simulink model "mcs_sim"  (R2014a)
settings: Solver=ode45  StartTime=0.0  StopTime=0.1  RelTol=1e-3
values from neighbouring files (symbols this model uses):
  mcs_sys = sys_class    [create_all_sys.m]
  sysr = ss(A_r,B_r,C_r,0)    [model_reduction.m]
undefined symbols (not defined in the file or in its folder): sysb, sysb_x0, sysr_x0
settings Model: Creator=UX31  LastModifiedBy=UX31

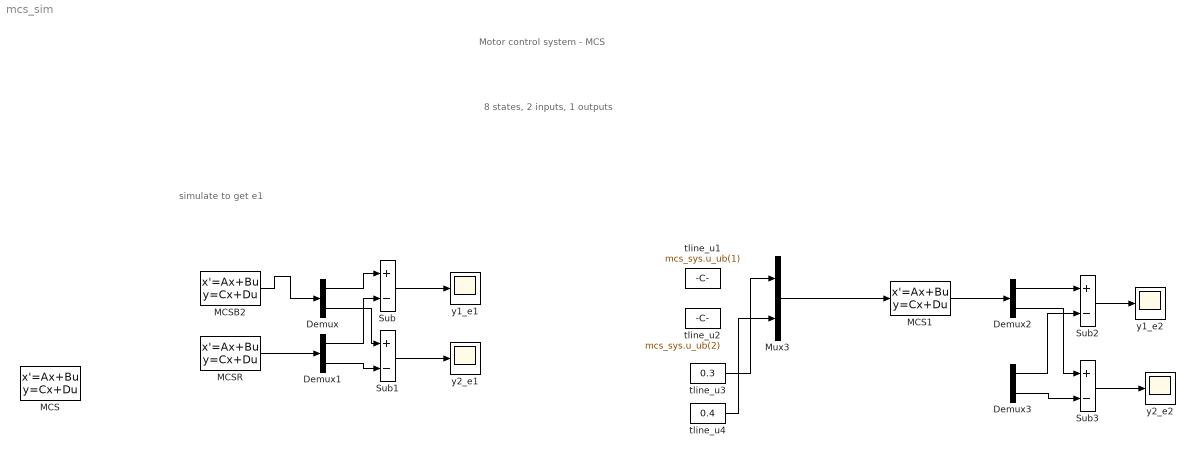
== system mcs_sim ==
  note: 8 states, 2 inputs, 1 outputs
  note: Motor control system - MCS
  note: simulate to get e1
  Demux{,1..3} (4 alike) : Demux  Outputs=2
  MCS : StateSpace  A=mcs_sys.sys.a  B=mcs_sys.sys.b  C=mcs_sys.sys.c  D=mcs_sys.sys.d  X0=mcs_sys.x0_lb
  MCS1 : StateSpace  A=mcs_sys.sys.a  B=mcs_sys.sys.b  C=mcs_sys.sys.c  D=mcs_sys.sys.d  X0=0
  MCSB2 : StateSpace  A=sysb.sys.a  B=sysb.sys.b  C=sysb.sys.c  D=sysb.sys.d  X0=sysb_x0
  MCSR : StateSpace  A=sysr.sys.a  B=sysr.sys.b  C=sysr.sys.c  D=sysr.sys.d  X0=sysr_x0
  Mux3 : Mux  Inputs=2
  Sub{,1..3} (4 alike) : Sum  Inputs=+-
  tline_u1 : Constant  Value=mcs_sys.u_ub(1)
  tline_u2 : Constant  Value=mcs_sys.u_ub(2)
  tline_u3 : Constant  Value=0.3
  tline_u4 : Constant  Value=0.4
  y1_e1 : Scope
      settings: TimeRange=0.04  YMin=0.06715860517435321  YMax=0.1151586051743532
  y1_e2 : Scope
      settings: SaveName=ScopeData2
  y2_e1 : Scope
      settings: SaveName=ScopeData12
  y2_e2 : Scope
      settings: SaveName=ScopeData3
  wires:
  Demux/1 -> Sub/1
  MCSR/1 -> Demux1/1
  Demux1/1 -> Sub/2
  Demux1/2 -> Sub1/2
  Demux/2 -> Sub1/1
  Sub1/1 -> y2_e1/1
  Sub/1 -> y1_e1/1
  Mux3/1 -> MCS1/1
  MCS1/1 -> Demux2/1
  Demux2/1 -> Sub2/1
  Demux3/1 -> Sub2/2
  Sub2/1 -> y1_e2/1
  Demux2/2 -> Sub3/1
  Demux3/2 -> Sub3/2
  Sub3/1 -> y2_e2/1
  tline_u3/1 -> Mux3/1
  tline_u4/1 -> Mux3/2
  MCSB2/1 -> Demux/1
